simulink model "Top_Level_Simulation_2019"  (R2019a)
settings: Solver=VariableStepAuto  StartTime=0.0  StopTime=stopTime  RelTol=1e-3
PreLoadFcn:
  | initializeParameters
InitFcn:
  | initializeParameters
StartFcn:
  | initializeParameters
undefined symbols (not defined in the file): bale, baleParam, cart, cartParam, contactGripper, floorParam, TsCtrl, X, Y, Z
libraries: sm_lib x229, nesl_utility x30, fl_lib x4, simulink x2, robotcorelib x2, robotmaniplib x2, Multibody_Multiphysics_Lib x2
(part 1 of 6)
settings Model: Creator=sabir  LastModifiedBy=sabir
settings DebuggingCC: UnconnectedInputMsg=none  UnconnectedOutputMsg=none  UnconnectedLineMsg=none
settings ModelReferenceCC: EnableRefExpFcnMdlSchedulingChecks=off
settings RTWCC: Description=Generic Real-Time Target

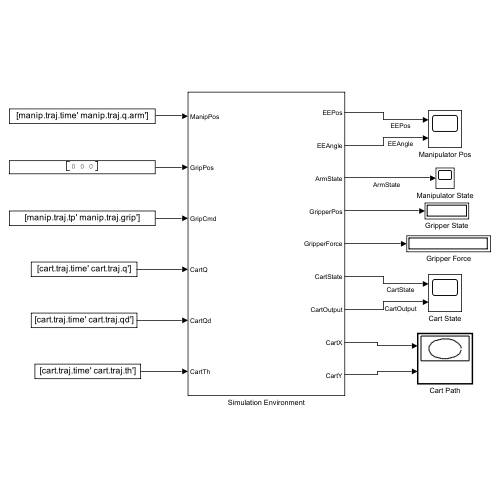
[thumbnail: Simulink's stored preview of the top-level diagram]
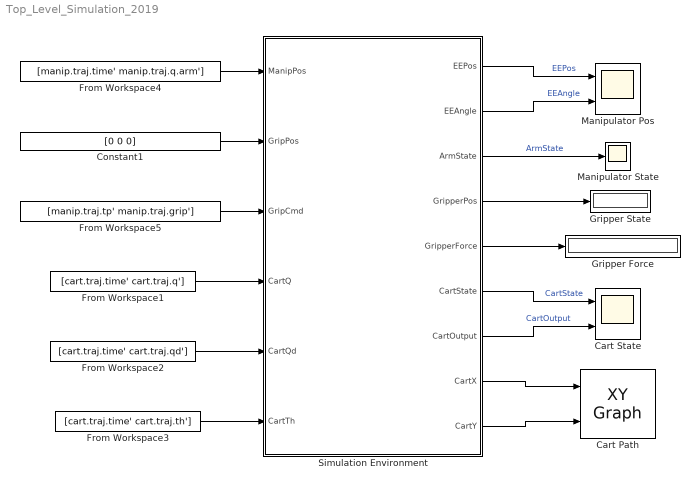
== system Top_Level_Simulation_2019 ==
  Cart Path : simulink/Sinks/XY Graph  xmin=-1  xmax=1  ymin=-1  ymax=1  st=-1
  Cart State : Scope  NumInputPorts=2
  Constant1 : Constant  Value=[0 0 0]
  From Workspace1 : FromWorkspace  VariableName=[cart.traj.time' cart.traj.q']  SampleTime=cart.traj.dt  OutputAfterFinalValue=Holding final value
  From Workspace2 : FromWorkspace  VariableName=[cart.traj.time' cart.traj.qd']  SampleTime=cart.traj.dt  OutputAfterFinalValue=Holding final value
  From Workspace3 : FromWorkspace  VariableName=[cart.traj.time' cart.traj.th']  SampleTime=cart.traj.dt  OutputAfterFinalValue=Holding final value
  From Workspace4 : FromWorkspace  VariableName=[manip.traj.time' manip.traj.q.arm']  SampleTime=-1  OutputAfterFinalValue=Holding final value
  From Workspace5 : FromWorkspace  VariableName=[manip.traj.tp' manip.traj.grip']  SampleTime=0.01  Interpolate=off  OutputAfterFinalValue=Setting to zero
  Gripper Force : Display
  Gripper State : Display
  Manipulator Pos : Scope  NumInputPorts=2
  Manipulator State : Scope
  Simulation Environment : Subsystem
  wires:
  From Workspace4/1 -> Simulation Environment/1(ManipPos)
  Constant1/1 -> Simulation Environment/2(GripPos)
  From Workspace5/1 -> Simulation Environment/3(GripCmd)
  From Workspace1/1 -> Simulation Environment/4(CartQ)
  From Workspace2/1 -> Simulation Environment/5(CartQd)
  From Workspace3/1 -> Simulation Environment/6(CartTh)
  Simulation Environment/1(EEPos) -> Manipulator Pos/1  "EEPos"
  Simulation Environment/2(EEAngle) -> Manipulator Pos/2  "EEAngle"
  Simulation Environment/3(ArmState) -> Manipulator State/1  "ArmState"
  Simulation Environment/4(GripperPos) -> Gripper State/1
  Simulation Environment/5(GripperForce) -> Gripper Force/1
  Simulation Environment/6(CartState) -> Cart State/1  "CartState"
  Simulation Environment/7(CartOutput) -> Cart State/2  "CartOutput"
  Simulation Environment/8(CartX) -> Cart Path/1
  Simulation Environment/9(CartY) -> Cart Path/2

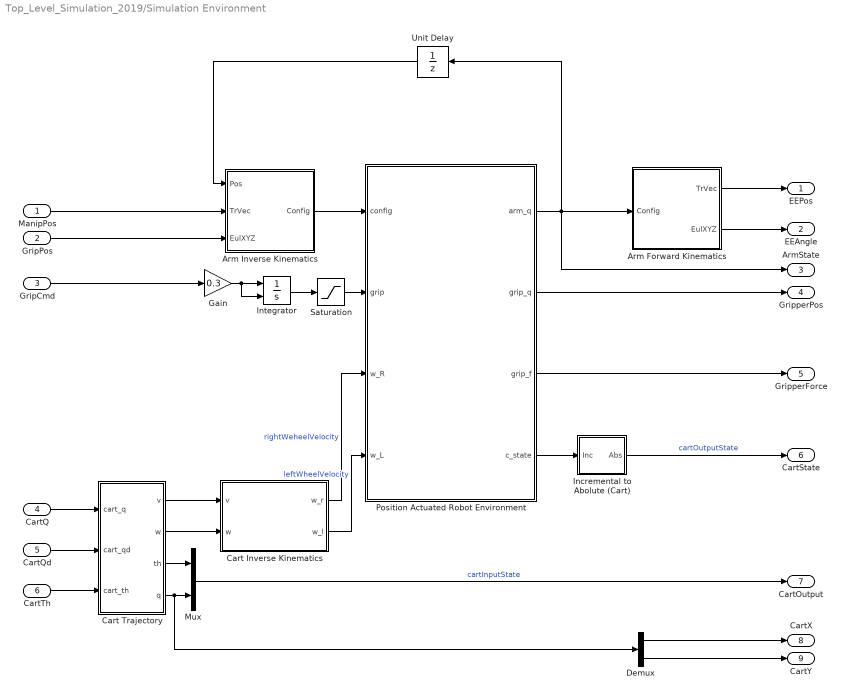
== system Top_Level_Simulation_2019/Simulation Environment ==
  ManipPos : Inport
  GripPos : Inport  Port=2
  GripCmd : Inport  Port=3
  CartQ : Inport  Port=4
  CartQd : Inport  Port=5
  CartTh : Inport  Port=6
  Arm Forward Kinematics : Subsystem
  Arm Inverse Kinematics : Subsystem
  Cart Inverse Kinematics : Subsystem
  Cart Trajectory : Subsystem
  Demux : Demux  Outputs=2
  Gain : Gain  Gain=0.3
  Incremental to Abolute (Cart) : Subsystem
  Integrator : Integrator  ExternalReset=falling
  Mux : Mux  Inputs=2
  Position Actuated Robot Environment : Subsystem  AutoFrameSizeCalculation=on
  Saturation : Saturate  UpperLimit=0.075  LowerLimit=0
  Unit Delay : UnitDelay  SampleTime=TsCtrl*10  HasFrameUpgradeWarning=on
  EEPos : Outport
  EEAngle : Outport  Port=2
  ArmState : Outport  Port=3
  GripperPos : Outport  Port=4
  GripperForce : Outport  Port=5
  CartState : Outport  Port=6
  CartOutput : Outport  Port=7
  CartX : Outport  Port=8
  CartY : Outport  Port=9
  wires:
  Arm Inverse Kinematics/1(Config) -> Position Actuated Robot Environment/1(config)
  Gain/1 -> Integrator/2, Integrator/1
  Integrator/1 -> Saturation/1
  Position Actuated Robot Environment/1(arm_q) -> ArmState/1, Arm Forward Kinematics/1(Config), Unit Delay/1
  Cart Trajectory/3(th) -> Mux/1
  Position Actuated Robot Environment/3(grip_f) -> GripperForce/1
  Cart Trajectory/2(w) -> Cart Inverse Kinematics/2(w)
  Cart Trajectory/1(v) -> Cart Inverse Kinematics/1(v)
  Saturation/1 -> Position Actuated Robot Environment/2(grip)
  GripPos/1 -> Arm Inverse Kinematics/3(EulXYZ)
  Unit Delay/1 -> Arm Inverse Kinematics/1(Pos)
  Cart Trajectory/4(q) -> Demux/1, Mux/2
  CartTh/1 -> Cart Trajectory/3(cart_th)
  Arm Forward Kinematics/2(EulXYZ) -> EEAngle/1
  Cart Inverse Kinematics/1(w_r) -> Position Actuated Robot Environment/3(w_R)  "rightWeheelVelocity"
  Position Actuated Robot Environment/4(c_state) -> Incremental to Abolute (Cart)/1(Inc)
  Cart Inverse Kinematics/2(w_l) -> Position Actuated Robot Environment/4(w_L)  "leftWheelVelocity"
  GripCmd/1 -> Gain/1
  CartQd/1 -> Cart Trajectory/2(cart_qd)
  CartQ/1 -> Cart Trajectory/1(cart_q)
  Demux/2 -> CartY/1
  Demux/1 -> CartX/1
  ManipPos/1 -> Arm Inverse Kinematics/2(TrVec)
  Arm Forward Kinematics/1(TrVec) -> EEPos/1
  Mux/1 -> CartOutput/1  "cartInputState"
  Incremental to Abolute (Cart)/1(Abs) -> CartState/1  "cartOutputState"
  Position Actuated Robot Environment/2(grip_q) -> GripperPos/1

== system Top_Level_Simulation_2019/Simulation Environment/Arm Forward Kinematics ==
  Config : Inport
  Coordinate Transformation Conversion : robotcorelib/Coordinate Transformation Conversion  InputRepresentation=Homogeneous Transformation  InputEulerSequence=ZYX  ShowTrVecInputPort=on  OutputRepresentation=Euler Angles  OutputEulerSequence=XYZ  ShowTrVecOutputPort=on  SimulateUsing=Interpreted execution
  Gain : Gain  Gain=-1
  Get Transform : robotmaniplib/Get Transform  RigidBodyTree=manipulator_tree  SourceBody=Base  TargetBody=Body7  SimulateUsing=Interpreted execution
  TrVec : Outport
  EulXYZ : Outport  Port=2
  wires:
  Get Transform/1 -> Coordinate Transformation Conversion/1
  Config/1 -> Get Transform/1
  Coordinate Transformation Conversion/2 -> Gain/1
  Gain/1 -> TrVec/1
  Coordinate Transformation Conversion/1 -> EulXYZ/1

== system Top_Level_Simulation_2019/Simulation Environment/Arm Inverse Kinematics ==
  Pos : Inport
  TrVec : Inport  Port=2
  EulXYZ : Inport  Port=3
  Constant2 : Constant  Value=[1 1 1 1 1 1]
  Coordinate Transformation Conversion : robotcorelib/Coordinate Transformation Conversion  InputRepresentation=Euler Angles  InputEulerSequence=XYZ  ShowTrVecInputPort=on  OutputRepresentation=Homogeneous Transformation  OutputEulerSequence=ZYX  ShowTrVecOutputPort=on  SimulateUsing=Code generation
  Inverse Kinematics : robotmaniplib/Inverse Kinematics  RigidBodyTree=manipulator_tree  EndEffector=Body7  ShowInfo=on  SolverName=BFGS Gradient Projection  EnforceJointLimits=on  MaxIterations=50  MaxTime=3  GradientTolerance=1e-7  SolutionTolerance=1e-6  StepTolerance=1e-12  ErrorChangeTolerance=1e-6  UseErrorDamping=on  DampingBias=0.0025  SimulateUsing=Code generation
  Transpose : Math  Operator=transpose  SaturateOnIntegerOverflow=on
  Config : Outport
  wires:
  Inverse Kinematics/1 -> Config/1
  Constant2/1 -> Inverse Kinematics/2
  Transpose/1 -> Inverse Kinematics/3
  EulXYZ/1 -> Coordinate Transformation Conversion/1
  TrVec/1 -> Coordinate Transformation Conversion/2
  Coordinate Transformation Conversion/1 -> Inverse Kinematics/1
  Pos/1 -> Transpose/1

== system Top_Level_Simulation_2019/Simulation Environment/Cart Inverse Kinematics ==
  v : Inport
  w : Inport  Port=2
  Mux : Mux  Inputs=2
  cartTraj2Signal : Subsystem
  w_r : Outport
  w_l : Outport  Port=2
  wires:
  w/1 -> Mux/2
  v/1 -> Mux/1
  Mux/1 -> cartTraj2Signal/1(u)
  cartTraj2Signal/1(w_r) -> w_r/1
  cartTraj2Signal/2(w_l) -> w_l/1

== system Top_Level_Simulation_2019/Simulation Environment/Cart Trajectory ==
  cart_q : Inport
  cart_qd : Inport  Port=2
  cart_th : Inport  Port=3
  Discrete Derivative : simulink/Discrete/Discrete Derivative  gainval=1.0  ICPrevScaledInput=0.0  OutMin=[]  OutMax=[]  OutDataType=fixdt(1, 16)  OutScaling=2^-10  DoSatur=off
  Gain : Gain  Gain=-1
  v : Outport
  w : Outport  Port=2
  th : Outport  Port=3
  q : Outport  Port=4
  wires:
  cart_th/1 -> th/1, Discrete Derivative/1
  cart_q/1 -> q/1
  cart_qd/1 -> v/1
  Discrete Derivative/1 -> Gain/1
  Gain/1 -> w/1

== system Top_Level_Simulation_2019/Simulation Environment/Incremental to Abolute (Cart) ==
  Inc : Inport
  Constant : Constant  Value=[cartParam.Initial.X cartParam.Initial.Y cartParam.Initial.Phase]
  Sum : Sum  Inputs=|++
  Abs : Outport
  wires:
  Constant/1 -> Sum/2
  Inc/1 -> Sum/1
  Sum/1 -> Abs/1

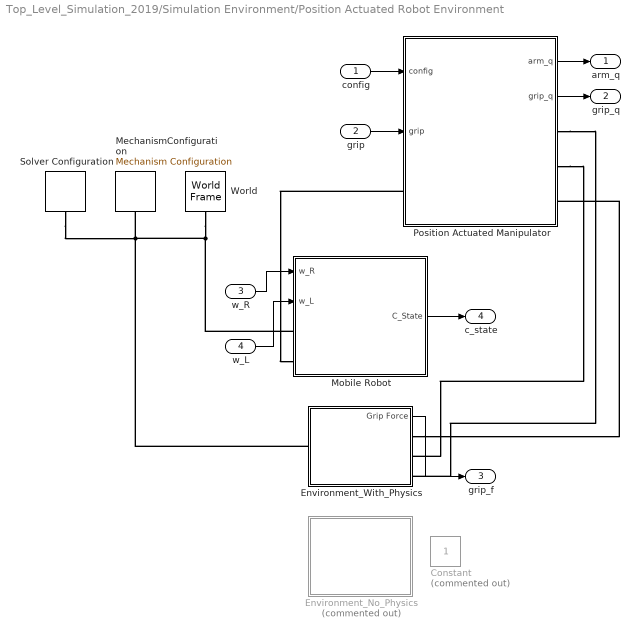
== system Top_Level_Simulation_2019/Simulation Environment/Position Actuated Robot Environment ==
  config : Inport
  grip : Inport  Port=2
  w_R : Inport  Port=3
  w_L : Inport  Port=4
  Constant : Constant  Commented=on
  Environment_No_Physics : Subsystem  Commented=on
  Environment_With_Physics : Subsystem  AutoFrameSizeCalculation=on
  MechanismConfiguration : sm_lib/Utilities/Mechanism Configuration  UniformGravity=Constant  GravityVector=[0 0 -9.80665]  GravityVectorUnits=m/s^2  LinearizationDelta=0.001  JointModeTransitionNonlinearIterations=2
  Mobile Robot : Subsystem
  Position Actuated Manipulator : Subsystem
  Solver Configuration : nesl_utility/Solver Configuration  PhysicalDomain=network_engine_domain  SubClassName=solver  LeftPortType=input  RightPortType=generic  Tones=[]  Harmonics=[]  SimulateNoise=off  Profile=off  UseLocalSampling=off  EnableSwitchedLinearOptims=on  FrequencyDomain=off  UseCCode=off  RelTol=0.001  AbsTol=0.001  MinStep=1e-09  ToWorkspace=off  RevertToSquareIcSolve=off  NumHomotopyIterations=100  PhasorMode=off  PhasorModeNumHarmonics=1  ConsistencySolver=NEWTON_XTOL_AFTER_FTOL  IndexReductionMethod=DerivativeReplacement  DoDC=off  ResidualTolerance=1e-09  ConsistencyTolSource=GLOBAL  ConsistencyAbsTol=0.001  ConsistencyRelTol=0.001  ConsistencyTolFactor=0.001  UseLocalSolver=off  LocalSolverChoice=NE_BACKWARD_EULER_ADVANCER  ResolveIndetEquations=on  FunctionEvalNumThread=1  LocalSolverSampleTime=0.001  DoFixedCost=off  MaxNonlinIter=3  MaxModeIter=2  ComputeImpulses=off  ImpulseIterations=2  LinearAlgebra=Sparse  LinearAlgebraNumThread=0  EquationFormulation=NE_TIME_EF  DelaysMemoryBudget=10240  AutomaticFiltering=on  FilteringTimeConstant=filterCoeff  PartitionStorageMethod=AS_NEEDED  PartitionMemoryBudget=1024  PartitionMethod=ROBUST
  World : sm_lib/Frames and Transforms/World Frame
  arm_q : Outport
  grip_q : Outport  Port=2
  grip_f : Outport  Port=3
  c_state : Outport  Port=4
  wires:
  grip/1 -> Position Actuated Manipulator/2(grip)
  Position Actuated Manipulator/1(arm_q) -> arm_q/1
  Position Actuated Manipulator/2(grip_q) -> grip_q/1
  w_R/1 -> Mobile Robot/1(w_R)
  Mobile Robot/1(C_State) -> c_state/1
  w_L/1 -> Mobile Robot/2(w_L)
  config/1 -> Position Actuated Manipulator/1(config)
  Environment_With_Physics/1(Grip Force) -> grip_f/1
  connections:
  Mobile Robot/LConn1 -- Environment_With_Physics/LConn1 -- Solver Configuration/RConn1 -- MechanismConfiguration/RConn1 -- World/RConn1
  Position Actuated Manipulator/LConn1 -- Mobile Robot/LConn2
  Position Actuated Manipulator/RConn2 -- Environment_With_Physics/RConn2
  Position Actuated Manipulator/RConn1 -- Environment_With_Physics/RConn3
  Environment_With_Physics/RConn1 -- Position Actuated Manipulator/RConn3

== system Top_Level_Simulation_2019/Simulation Environment/Cart Inverse Kinematics/cartTraj2Signal ==
  u : Inport
  Constant : Constant  Value=cartParam.TireRadius
  Constant1 : Constant  Value=cartParam.DistanceBwTires
  cartTraj2Signal : MATLAB Function  TreatAsAtomicUnit=on
  w_r : Outport
  w_l : Outport  Port=2
  wires:
  cartTraj2Signal/2(w_l) -> w_l/1
  Constant/1 -> cartTraj2Signal/2(r)
  Constant1/1 -> cartTraj2Signal/3(b)
  u/1 -> cartTraj2Signal/1(u)
  cartTraj2Signal/1(w_r) -> w_r/1

== system Top_Level_Simulation_2019/Simulation Environment/Position Actuated Robot Environment/Environment_No_Physics ==
  Bale1 : sm_lib/Body Elements/Solid  GraphicAmbientColor=[0.15 0.15 0.15 1.0]  BasedOnType=Mass  CenterOfMass=[0 0 0]  CenterOfMassUnits=m  GraphicDiffuseColor=[0.8 0.6 0.0]  CylinderLength=baleParam.Length  CylinderLengthUnits=m  CylinderRadius=baleParam.Radius  CylinderRadiusUnits=m  Density=1000  DensityUnits=kg/m^3  DoExposeReferenceFrame=on  GraphicEmissiveColor=[0.0 0.0 0.0 1.0]  ExportEntireGeometry=off  SerializedFrames=<Frames/>  MarkerShape=Sphere  MarkerSize=10  GraphicType=FromGeometry  InertiaType=CalculateFromGeometry  Mass=baleParam.Mass  MassUnits=kg  MomentsOfInertia=[1 1 1]  MomentsOfInertiaUnits=kg*m^2  GraphicOpacity=1.0  ProductsOfInertia=[0 0 0]  ProductsOfInertiaUnits=kg*m^2  GraphicShininess=75  GraphicSpecularColor=[0.5 0.5 0.5 1.0]  GraphicVisPropType=SimpleVisualProperties  GeometryShape=Cylinder
  Bale2 : sm_lib/Body Elements/Solid  GraphicAmbientColor=[0.15 0.15 0.15 1.0]  BasedOnType=Mass  CenterOfMass=[0 0 0]  CenterOfMassUnits=m  GraphicDiffuseColor=[0.8 0.6 0.0]  CylinderLength=baleParam.Length  CylinderLengthUnits=m  CylinderRadius=baleParam.Radius  CylinderRadiusUnits=m  Density=1000  DensityUnits=kg/m^3  DoExposeReferenceFrame=on  GraphicEmissiveColor=[0.0 0.0 0.0 1.0]  ExportEntireGeometry=off  SerializedFrames=<Frames/>  MarkerShape=Sphere  MarkerSize=10  GraphicType=FromGeometry  InertiaType=CalculateFromGeometry  Mass=baleParam.Mass  MassUnits=kg  MomentsOfInertia=[1 1 1]  MomentsOfInertiaUnits=kg*m^2  GraphicOpacity=1.0  ProductsOfInertia=[0 0 0]  ProductsOfInertiaUnits=kg*m^2  GraphicShininess=75  GraphicSpecularColor=[0.5 0.5 0.5 1.0]  GraphicVisPropType=SimpleVisualProperties  GeometryShape=Cylinder
  Drop : sm_lib/Body Elements/Solid  GraphicAmbientColor=[0.15 0.15 0.15 1.0]  BasedOnType=Density  BrickDimensions=[2 1.3 1.0E-4]  BrickDimensionsUnits=m  CenterOfMass=[0 0 0]  CenterOfMassUnits=m  GraphicDiffuseColor=[0.4 1.0 0.8]  Density=1000  DensityUnits=kg/m^3  DoExposeReferenceFrame=off  GraphicEmissiveColor=[0.0 0.0 0.0 1.0]  ExportEntireGeometry=off  SerializedFrames=<Frames><Frame><Id>Frame1</Id><Value><Name>R</Name><Origin><Source>GeometricFeature</Source><FeatureName>+y +z curve</FeatureName></Origin><PrimaryAxis><DefinedDirection>+Z</DefinedDirection><Source>ReferenceFrame</Source><SourceDirection>+Z</SourceDirection><FeatureName></FeatureName></PrimaryAxis><SecondaryAxis><DefinedDirection>+X</DefinedDirection><Source>ReferenceFrame</Source><SourceDirection>+X</SourceDirection><FeatureName></FeatureName></SecondaryAxis></Value></Frame></Frames>  MarkerShape=Sphere  MarkerSize=10  GraphicType=FromGeometry  InertiaType=CalculateFromGeometry  Mass=1  MassUnits=kg  MomentsOfInertia=[1 1 1]  MomentsOfInertiaUnits=kg*m^2  GraphicOpacity=0.6  ProductsOfInertia=[0 0 0]  ProductsOfInertiaUnits=kg*m^2  GraphicShininess=75  GraphicSpecularColor=[0.5 0.5 0.5 1.0]  GraphicVisPropType=SimpleVisualProperties  GeometryShape=Brick
  Floor : sm_lib/Body Elements/Solid  GraphicAmbientColor=[0.15 0.15 0.15 1.0]  BasedOnType=Density  BrickDimensions=[floorParam.X floorParam.Y 1.0E-4]  BrickDimensionsUnits=m  CenterOfMass=[0 0 0]  CenterOfMassUnits=m  GraphicDiffuseColor=[0.6 1.0 0.6]  Density=1000  DensityUnits=kg/m^3  DoExposeReferenceFrame=off  GraphicEmissiveColor=[0.0 0.0 0.0 1.0]  ExportEntireGeometry=off  SerializedFrames=<Frames><Frame><Id>Frame1</Id><Value><Name>R</Name><Origin><Source>GeometricFeature</Source><FeatureName>-x -y +z point</FeatureName></Origin><PrimaryAxis><DefinedDirection>+Z</DefinedDirection><Source>ReferenceFrame</Source><SourceDirection>+Z</SourceDirection><FeatureName></FeatureName></PrimaryAxis><SecondaryAxis><DefinedDirection>+X</DefinedDirection><Source>ReferenceFrame</Source><SourceDirection>+X</SourceDirection><FeatureName></FeatureName></SecondaryAxis></Value></Frame></Frames>  MarkerShape=Sphere  MarkerSize=10  GraphicType=FromGeometry  InertiaType=CalculateFromGeometry  Mass=1  MassUnits=kg  MomentsOfInertia=[1 1 1]  MomentsOfInertiaUnits=kg*m^2  GraphicOpacity=0.6  ProductsOfInertia=[0 0 0]  ProductsOfInertiaUnits=kg*m^2  GraphicShininess=75  GraphicSpecularColor=[0.5 0.5 0.5 1.0]  GraphicVisPropType=SimpleVisualProperties  GeometryShape=Brick
  Rigid Transform1 : sm_lib/Frames and Transforms/Rigid Transform  TranslationMethod=Cartesian  TranslationStandardOffset=0  TranslationStandardOffsetUnits=m  TranslationStandardAxis=+Z  TranslationCartesianOffset=[bale.One.X bale.One.Y baleParam.Radius]  TranslationCartesianOffsetUnits=m  TranslationROffset=0  TranslationROffsetUnits=m  TranslationZOffset=0  TranslationZOffsetUnits=m  TranslationThetaOffset=0  TranslationThetaOffsetUnits=deg  RotationMethod=RotationSequence  RotationAngleUnits=deg  RotationStandardAxis=+Y  RotationAngle=-90  RotationArbitraryAxis=[0 0 1]  FollAlignAxisA=+X  BaseAlignAxisA=+Y  FollAlignAxisB=+Y  BaseAlignAxisB=+Z  RotationSequenceAxes=BaseAxes  RotationSequence=XYZ  RotationSequenceAngles=[bale.One.Rot]  RotationSequenceAnglesUnits=deg  RotationMatrix=[1 0 0; 0 1 0; 0 0 1]  Quaternion=[1 0 0 0]
  Rigid Transform2 : sm_lib/Frames and Transforms/Rigid Transform  TranslationMethod=Cartesian  TranslationStandardOffset=0  TranslationStandardOffsetUnits=m  TranslationStandardAxis=+Z  TranslationCartesianOffset=[bale.Two.X bale.Two.Y baleParam.Radius]  TranslationCartesianOffsetUnits=m  TranslationROffset=0  TranslationROffsetUnits=m  TranslationZOffset=0  TranslationZOffsetUnits=m  TranslationThetaOffset=0  TranslationThetaOffsetUnits=deg  RotationMethod=RotationSequence  RotationAngleUnits=deg  RotationStandardAxis=+Y  RotationAngle=-90  RotationArbitraryAxis=[0 0 1]  FollAlignAxisA=+X  BaseAlignAxisA=+Y  FollAlignAxisB=+Y  BaseAlignAxisB=+Z  RotationSequenceAxes=BaseAxes  RotationSequence=XYZ  RotationSequenceAngles=[bale.Two.Rot]  RotationSequenceAnglesUnits=deg  RotationMatrix=[1 0 0; 0 1 0; 0 0 1]  Quaternion=[1 0 0 0]
  Rigid Transform3 : sm_lib/Frames and Transforms/Rigid Transform  TranslationMethod=Cartesian  TranslationStandardOffset=0  TranslationStandardOffsetUnits=m  TranslationStandardAxis=+Z  TranslationCartesianOffset=[10 0 1.5]  TranslationCartesianOffsetUnits=m  TranslationROffset=0  TranslationROffsetUnits=m  TranslationZOffset=0  TranslationZOffsetUnits=m  TranslationThetaOffset=0  TranslationThetaOffsetUnits=deg  RotationMethod=None  RotationAngleUnits=deg  RotationStandardAxis=+Y  RotationAngle=-90  RotationArbitraryAxis=[0 0 1]  FollAlignAxisA=+X  BaseAlignAxisA=+Y  FollAlignAxisB=+Y  BaseAlignAxisB=+Z  RotationSequenceAxes=FollowerAxes  RotationSequence=XYX  RotationSequenceAngles=[0 0 0]  RotationSequenceAnglesUnits=deg  RotationMatrix=[1 0 0; 0 1 0; 0 0 1]  Quaternion=[1 0 0 0]
  Rigid Transform7 : sm_lib/Frames and Transforms/Rigid Transform  TranslationMethod=Cartesian  TranslationStandardOffset=0  TranslationStandardOffsetUnits=m  TranslationStandardAxis=+Z  TranslationCartesianOffset=[0.7 0.7 0]  TranslationCartesianOffsetUnits=m  TranslationROffset=0  TranslationROffsetUnits=m  TranslationZOffset=0  TranslationZOffsetUnits=m  TranslationThetaOffset=0  TranslationThetaOffsetUnits=deg  RotationMethod=StandardAxis  RotationAngleUnits=deg  RotationStandardAxis=+Z  RotationAngle=135  RotationArbitraryAxis=[0 0 1]  FollAlignAxisA=+X  BaseAlignAxisA=+Y  FollAlignAxisB=+Y  BaseAlignAxisB=+Z  RotationSequenceAxes=FollowerAxes  RotationSequence=XYX  RotationSequenceAngles=[0 0 0]  RotationSequenceAnglesUnits=deg  RotationMatrix=[1 0 0; 0 1 0; 0 0 1]  Quaternion=[1 0 0 0]
  farmer_guy : Subsystem
  World : PMIOPort  Side=Left
  connections:
  Bale2/RConn1 -- Rigid Transform2/RConn1
  Floor/LConn1 -- Rigid Transform7/LConn1 -- Rigid Transform3/LConn1 -- World/RConn1 -- Rigid Transform2/LConn1 -- Rigid Transform1/LConn1
  Bale1/RConn1 -- Rigid Transform1/RConn1
  Drop/LConn1 -- Rigid Transform3/RConn1
  Rigid Transform7/RConn1 -- farmer_guy/LConn1
